simulink model "VIENA_testeJF"  (R2020a)
settings: Solver=VariableStepAuto  StartTime=0.0  StopTime=100  FixedStep=dt  MaxStep=1e-4  RelTol=1e-4
values from neighbouring files (symbols this model uses):
  g = 9.8    [checkSlip.m]    (also in globalDef.m)
  lr = 0.06709e-3    (= 6.709e-05)    [createVParam.m]    (also in vehicleParameters.mat)
  M = 900    [globalDef.m]
  pdelta = simU(i,2)    [main2.m]
  x0 = ocp.get('x', 1)    [main2.m]
undefined symbols (not defined in the file or in its folder): lf, psi0, Steering, y0
libraries: simulink_extras x1, spsEdgeDetectorLib x1, autolibshared x1
settings Model: Creator=João Fernandes  LastModifiedBy=jpfin
settings DataIOCC: ReturnWorkspaceOutputs=off
settings DebuggingCC: ArithmeticOperatorsInVariantConditions=warning
settings SFSimCC: SimUseLocalCustomCode=off  CustomCodeUndefinedFunction=UseInterfaceOnly
settings RTWCC: RTWUseLocalCustomCode=off

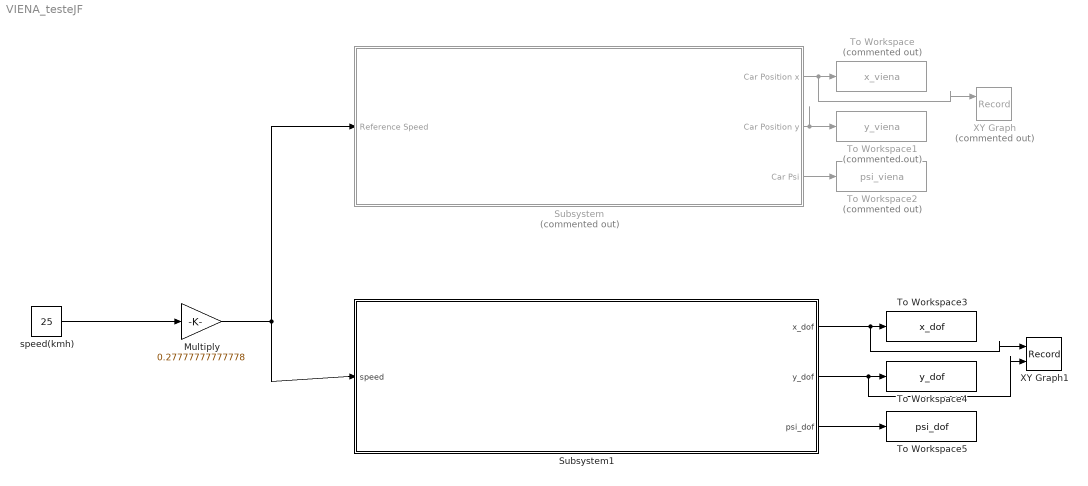
== system VIENA_testeJF ==
  Multiply : Gain  Gain=0.27777777777778
  Subsystem : Subsystem  Commented=on
      mask Display: image('vienalogo.jpg');
  Subsystem1 : Subsystem
  To Workspace : ToWorkspace  Commented=on  VariableName=x_viena  SaveFormat=Timeseries  SampleTime=-1
  To Workspace1 : ToWorkspace  Commented=on  VariableName=y_viena  SaveFormat=Timeseries  SampleTime=-1
  To Workspace2 : ToWorkspace  Commented=on  VariableName=psi_viena  SaveFormat=Timeseries  SampleTime=-1
  To Workspace3 : ToWorkspace  VariableName=x_dof  SaveFormat=Timeseries  SampleTime=-1
  To Workspace4 : ToWorkspace  VariableName=y_dof  SaveFormat=Timeseries  SampleTime=-1
  To Workspace5 : ToWorkspace  VariableName=psi_dof  SaveFormat=Timeseries  SampleTime=-1
  XY Graph : Record  Commented=on  Layout=[1 1]
  XY Graph1 : Record  Layout=[1 1]
  speed(kmh) : Constant  Value=25
  wires:
  Subsystem/1(Car Position x) -> XY Graph/1, To Workspace/1
  Subsystem/2(Car Position y) -> To Workspace1/1
  Subsystem/3(Car Psi) -> To Workspace2/1
  Subsystem1/1(x_dof) -> XY Graph1/1, To Workspace3/1
  Subsystem1/2(y_dof) -> XY Graph1/2, To Workspace4/1
  Subsystem1/3(psi_dof) -> To Workspace5/1
  Multiply/1 -> Subsystem1/1(speed), Subsystem/1(Reference Speed)
  speed(kmh)/1 -> Multiply/1

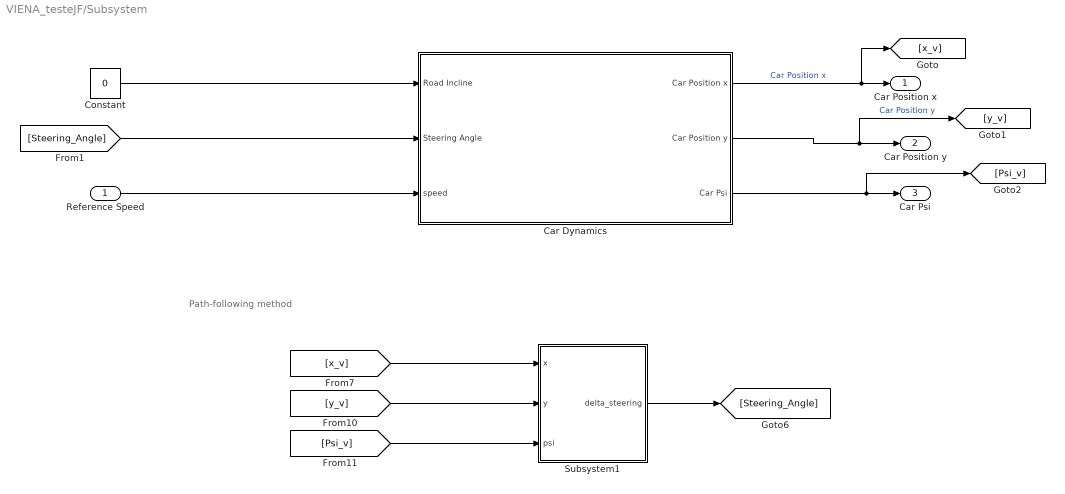
== system VIENA_testeJF/Subsystem ==
  note: Path-following method
  Reference Speed : Inport
  Car Dynamics : Subsystem
  Constant : Constant  Value=0
  Subsystem1 : Subsystem
  Car Position x : Outport  VectorParamsAs1DForOutWhenUnconnected=off
  Car Position y : Outport  Port=2  VectorParamsAs1DForOutWhenUnconnected=off
  Car Psi : Outport  Port=3  VectorParamsAs1DForOutWhenUnconnected=off
  wires:
  Constant/1 -> Car Dynamics/1(Road Incline)
  Car Dynamics/1(Car Position x) -> [x_v], Car Position x/1  "Car Position x"
  [Steering_Angle] -> Car Dynamics/2(Steering Angle)
  Car Dynamics/2(Car Position y) -> [y_v], Car Position y/1  "Car Position y"
  Car Dynamics/3(Car Psi) -> [Psi_v], Car Psi/1
  Reference Speed/1 -> Car Dynamics/3(speed)
  [y_v] -> Subsystem1/2(y)
  [x_v] -> Subsystem1/1(x)
  [Psi_v] -> Subsystem1/3(psi)
  Subsystem1/1(delta_steering) -> [Steering_Angle]

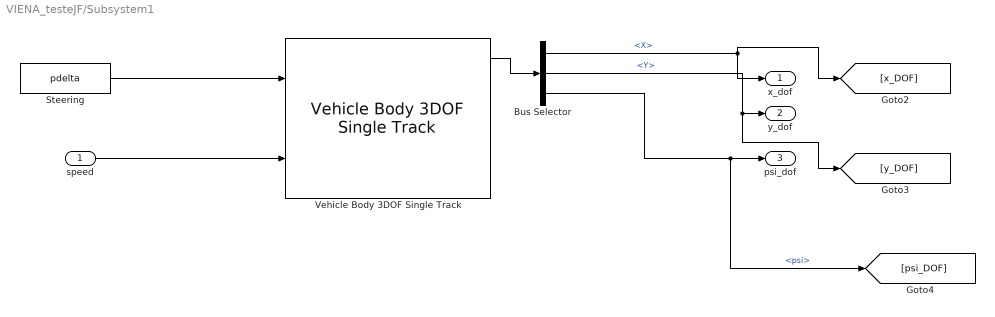
== system VIENA_testeJF/Subsystem1 ==
  speed : Inport
  Bus Selector : BusSelector  OutputSignals=InertFrm.Cg.Disp.X,InertFrm.Cg.Disp.Y,InertFrm.Cg.Ang.psi
  Steering : Constant  Value=pdelta
  Vehicle Body 3DOF Single Track : autolibshared/Vehicle Body 3DOF Single Track  trackMode=Single (bicycle)  inputMode=External longitudinal velocity  frontSteerMode=on  rearSteerMode=off  windMode=off  muMode=off  extFMode=off  extMMode=off  extXo=off  extpsio=off  extxdoto=off  extro=off  extYo=off  extTamb=off  extydoto=off  aMode=2  NF=2  NR=2  m=800  a=3.23/2  b=3.23/2  h=0.35  X_o=0  xdot_o=0  CalphaMode=off  sigmaMode=on  d=0  w=[1.4,1.4]  Cy_f=12e3  Cy_r=11e3  sigma_f=.1  sigma_r=.1  alpha_f_brk=[-.1 .1]  Cy_f_data=[-9e3 9e3]  alpha_r_brk=[-.1 .1]  Cy_r_data=[-9e3 9e3]  Y_o=0  ydot_o=0  Izz=84.55  psi_o=0  r_o=0  Af=A  Cd=Cd  Cl=.1  Cpm=.1  beta_w=[0 0.01:0.01:0.3]  Cs=[0 0.01:0.01:0.3]  Cym=[0 1e-6:0.01:0.3]  Pabs=101325  Tair=273  g=9.81  mu=1  xdot_tol=.01  Fznom=M*g  Fxtire_sat=7e4  Fytire_sat=7e4  longOff=0  latOff=0  vertOff=0  wrapAng=off
      settings: SourceProductBaseCode=PW,MT,VE,VP
  x_dof : Outport
  y_dof : Outport  Port=2
  psi_dof : Outport  Port=3
  wires:
  Steering/1 -> Vehicle Body 3DOF Single Track/1
  speed/1 -> Vehicle Body 3DOF Single Track/2
  Bus Selector/2 -> [y_DOF], y_dof/1  "<Y>"
  Vehicle Body 3DOF Single Track/1 -> Bus Selector/1
  Bus Selector/1 -> x_dof/1, [x_DOF]  "<X>"
  Bus Selector/3 -> [psi_DOF], psi_dof/1  "<psi>"

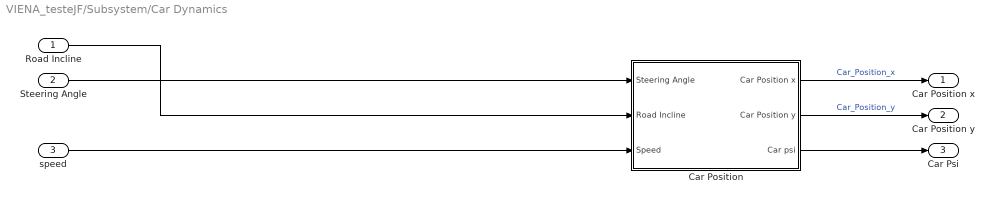
== system VIENA_testeJF/Subsystem/Car Dynamics ==
  Road Incline : Inport
  Steering Angle : Inport  Port=2
  speed : Inport  Port=3
  Car Position : Subsystem
  Car Position x : Outport  VectorParamsAs1DForOutWhenUnconnected=off
  Car Position y : Outport  Port=2  VectorParamsAs1DForOutWhenUnconnected=off
  Car Psi : Outport  Port=3  VectorParamsAs1DForOutWhenUnconnected=off
  wires:
  speed/1 -> Car Position/3(Speed)
  Steering Angle/1 -> Car Position/1(Steering Angle)
  Car Position/2(Car Position y) -> Car Position y/1  "Car_Position_y"
  Road Incline/1 -> Car Position/2(Road Incline)
  Car Position/1(Car Position x) -> Car Position x/1  "Car_Position_x"
  Car Position/3(Car psi) -> Car Psi/1

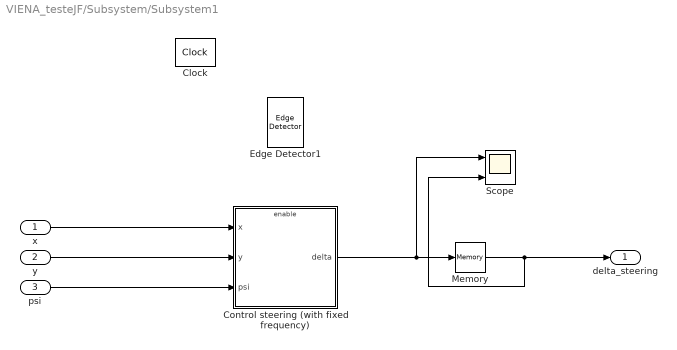
== system VIENA_testeJF/Subsystem/Subsystem1 ==
  x : Inport
  y : Inport  Port=2
  psi : Inport  Port=3
  Clock : simulink_extras/Flip Flops/Clock  period=dt
  Control steering (with fixed frequency) : Subsystem  TreatAsAtomicUnit=on
  Edge Detector1 : spsEdgeDetectorLib/Edge Detector  model=Rising  ic=0  Ts=0
      settings: LibrarySourceBlock=sps_lib/Control/Edge Detector
  Memory : Memory
  Scope : Scope  NumInputPorts=3
  delta_steering : Outport  VectorParamsAs1DForOutWhenUnconnected=off
  wires:
  ? -> Control steering (with fixed frequency)/Enable, Scope/2
  ? -> ?
  x/1 -> Control steering (with fixed frequency)/1(x)
  y/1 -> Control steering (with fixed frequency)/2(y)
  psi/1 -> Control steering (with fixed frequency)/3(psi)
  Control steering (with fixed frequency)/1(delta) -> Memory/1, Scope/1
  Memory/1 -> Scope/3, delta_steering/1

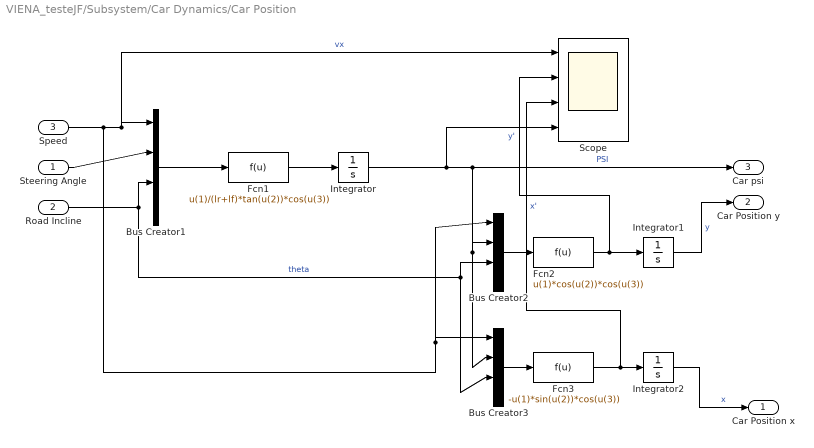
== system VIENA_testeJF/Subsystem/Car Dynamics/Car Position ==
  Steering Angle : Inport
  Road Incline : Inport  Port=2
  Speed : Inport  Port=3
  Bus Creator1 : BusCreator  Inputs=3
  Bus Creator2 : BusCreator  Inputs=3
  Bus Creator3 : BusCreator  Inputs=3
  Fcn1 : Fcn  Expr=u(1)/(lr+lf)*tan(u(2))*cos(u(3))
  Fcn2 : Fcn  Expr=u(1)*cos(u(2))*cos(u(3))
  Fcn3 : Fcn  Expr=-u(1)*sin(u(2))*cos(u(3))
  Integrator : Integrator  InitialCondition=psi0
  Integrator1 : Integrator  InitialCondition=y0
  Integrator2 : Integrator  InitialCondition=x0
  Scope : Scope  NumInputPorts=4
  Car Position x : Outport  VectorParamsAs1DForOutWhenUnconnected=off
  Car Position y : Outport  Port=2  VectorParamsAs1DForOutWhenUnconnected=off
  Car psi : Outport  Port=3  VectorParamsAs1DForOutWhenUnconnected=off
  wires:
  Integrator1/1 -> Car Position y/1  "y"
  Integrator2/1 -> Car Position x/1  "x"
  Road Incline/1 -> Bus Creator3/3, Bus Creator2/3, Bus Creator1/3  "theta"
  Bus Creator1/1 -> Fcn1/1
  Fcn1/1 -> Integrator/1
  Bus Creator2/1 -> Fcn2/1
  Speed/1 -> Bus Creator2/1, Bus Creator3/1, Scope/1, Bus Creator1/1  "vx"
  Fcn2/1 -> Scope/2, Integrator1/1  "y'"
  Fcn3/1 -> Scope/3, Integrator2/1  "x'"
  Integrator/1 -> Car psi/1, Bus Creator3/2, Bus Creator2/2, Scope/4  "PSI"
  Bus Creator3/1 -> Fcn3/1
  Steering Angle/1 -> Bus Creator1/2

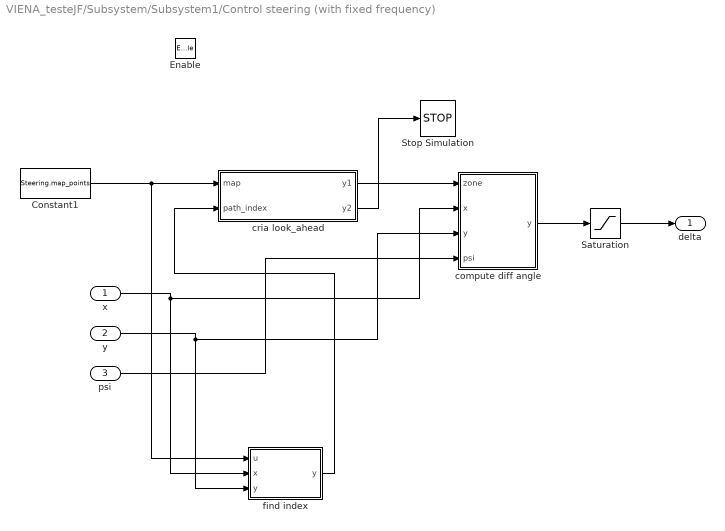
== system VIENA_testeJF/Subsystem/Subsystem1/Control steering (with fixed frequency) ==
  x : Inport
  y : Inport  Port=2
  psi : Inport  Port=3
  Enable : EnablePort
  Constant1 : Constant  Value=Steering.map_points  VectorParams1D=off
  Saturation : Saturate  UpperLimit=28*pi/180  LowerLimit=-28*pi/180
  Stop Simulation : Stop
  compute diff angle : MATLAB Function  TreatAsAtomicUnit=on
  cria look_ahead : MATLAB Function  TreatAsAtomicUnit=on
  find index : MATLAB Function  TreatAsAtomicUnit=on
  delta : Outport  VectorParamsAs1DForOutWhenUnconnected=off
  wires:
  x/1 -> compute diff angle/2(x), find index/2(x)
  y/1 -> compute diff angle/3("y "), find index/3("y ")
  Constant1/1 -> cria look_ahead/1(map), find index/1(u)
  find index/1(y) -> cria look_ahead/2(path_index)
  cria look_ahead/2(y2) -> Stop Simulation/1
  compute diff angle/1(y) -> Saturation/1
  cria look_ahead/1(y1) -> compute diff angle/1(zone)
  psi/1 -> compute diff angle/4(psi)
  Saturation/1 -> delta/1

== matlab function VIENA_testeJF/Subsystem/Subsystem1/Control steering (with fixed frequency)/cria look_ahead ==
  data: map input; y1 output; y2 output; path_index input
function [y1,y2] = fcn(map,path_index)

coder.extrinsic('vecnorm')

y2=0;
path_look_ahead=3;
N=length(map);

window = zeros(path_look_ahead+1,2);

for i=1:path_look_ahead+1
    if path_index+i-1>N
        window(i,:)=map(min(path_index+i-1,N),:);
    else
        window(i,:)=map(path_index+i-1,:);
    end
    
end

y1=window;

if path_index==N
    y2=1;
end

== matlab function VIENA_testeJF/Subsystem/Subsystem1/Control steering (with fixed frequency)/compute diff angle ==
  data: zone input; y output; x input; y input; psi input
function y = fcn(zone,x,y,psi)

car_direction_vector=[-sin(psi) cos(psi)];
look_ahead_vector=[(zone(end,1)-x),zone(end,2)-y];
angle_car = atan2(car_direction_vector(2),car_direction_vector(1));
angle_look_ahead = atan2(look_ahead_vector(2),look_ahead_vector(1));



angle_diff = (angle_look_ahead-angle_car);
while angle_diff>pi
    angle_diff=angle_diff-2*pi;
end
while angle_diff<-pi
    angle_diff=angle_diff+2*pi;
end
y= angle_diff;

== matlab function VIENA_testeJF/Subsystem/Subsystem1/Control steering (with fixed frequency)/find index ==
  data: u input; y output; x input; y input
function y = fcn(u,x,y)

coder.extrinsic('vecnorm')
map=u;

[~, path_index]=min(vecnorm(map-repmat([x y],length(map),1),2,2));

y= path_index;
